simulink model "Challenge1_2"  (R2020b)
settings: Solver=VariableStepAuto  StartTime=0.0  StopTime=10.0  RelTol=1e-3
settings Model: Creator=jimd  LastModifiedBy=jimd

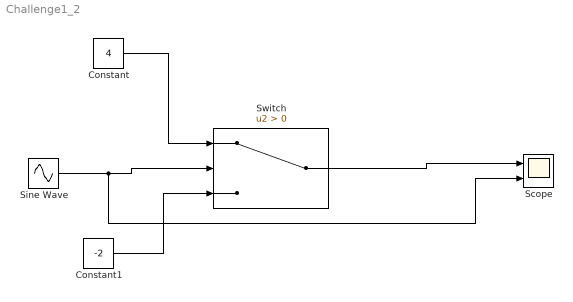
== system Challenge1_2 ==
  Constant : Constant  Value=4
  Constant1 : Constant  Value=-2
  Scope : Scope  NumInputPorts=2
  Sine Wave : Sin  SampleTime=0
  Switch : Switch  Criteria=u2 > Threshold
  wires:
  Constant/1 -> Switch/1
  Sine Wave/1 -> Scope/2, Switch/2
  Constant1/1 -> Switch/3
  Switch/1 -> Scope/1
